simulink model "ex4_5"  (R2020b)
settings: Solver=VariableStepAuto  StartTime=0.0  StopTime=0.04096  RelTol=1e-3
libraries: dspsrcs4 x1
settings Model: Creator=seojoon  LastModifiedBy=seojoon

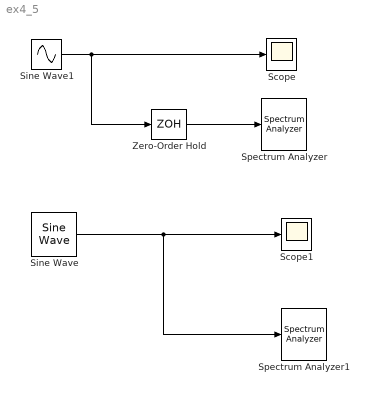
== system ex4_5 ==
  Scope : Scope
  Scope1 : Scope
  Sine Wave : dspsrcs4/Sine Wave  Amplitude=10  Frequency=1000  Phase=0  SampleMode=Discrete  OutComplex=Real  CompMethod=Trigonometric fcn  TableSize=Speed  SampleTime=1e-5  SamplesPerFrame=1  ResetState=Restart at time zero  OutputFrames=off  dataType=double  wordLen=16  udDataType=sfix(16)  fracBitsMode=Best precision  numFracBits=15  OutDataTypeStr=double  LastOutDataTypeStr=double
  Sine Wave1 : Sin  Amplitude=10  Frequency=2*pi*1000  SampleTime=0
  Spectrum Analyzer : SpectrumAnalyzer
  Spectrum Analyzer1 : SpectrumAnalyzer
  Zero-Order Hold : ZeroOrderHold  SampleTime=1e-5
  wires:
  Sine Wave1/1 -> Zero-Order Hold/1, Scope/1
  Zero-Order Hold/1 -> Spectrum Analyzer/1
  Sine Wave/1 -> Spectrum Analyzer1/1, Scope1/1
